simulink model "Lab6_Ris_2_20"  (Simulink 10.2)
settings: Solver=VariableStepAuto  StartTime=0.0  StopTime=10.0  RelTol=1e-3
undefined symbols (not defined in the file): dvbs2ldpc
libraries: commdigbbndam3 x5, commblkcod2 x3, commsink2 x2, commchan3 x1, commrandsrc3 x1, commutil2 x1
settings Model: Creator=Newtr  LastModifiedBy=Newtr
settings DataIOCC: SaveFormat=Dataset  SignalLoggingSaveFormat=Dataset  ReturnWorkspaceOutputs=on
settings OptimizationCC: LifeSpan=auto
settings DebuggingCC: UnderspecifiedInitializationDetection=Simplified  MergeDetectMultiDrivingBlocksExec=error  FcnCallInpInsideContextMsg=error  SFUnexpectedBacktrackingDiag=error  SFNoUnconditionalDefaultTransitionDiag=error  SFExecutionAtInitializationDiag=warning  ArithmeticOperatorsInVariantConditions=error
settings HardwareCC: ProdBitPerPointer=64  ProdBitPerSizeT=64  ProdBitPerPtrDiffT=64  ProdLargestAtomicFloat=Float  ProdIntDivRoundTo=Zero  ProdEndianess=LittleEndian  ProdWordSize=64  ProdHWDeviceType=Intel->x86-64 (Windows64)
settings ModelReferenceCC: PropagateSignalLabelsOutOfModel=on
settings SFSimCC: SimUseLocalCustomCode=on  CustomCodeUndefinedFunction=FilterOut
settings RTWCC: RTWUseLocalCustomCode=on
settings CodeAppCC: StateflowObjectComments=off
settings GRTTargetCC: TargetLangStandard=C99 (ISO)  CombineOutputUpdateFcns=on  GRTInterface=off
settings ConfigComp: CovMetricSettings=dwe  CovSaveCumulativeToWorkspaceVar=off  CovSaveSingleToWorkspaceVar=off  CovExternalEMLEnable=on

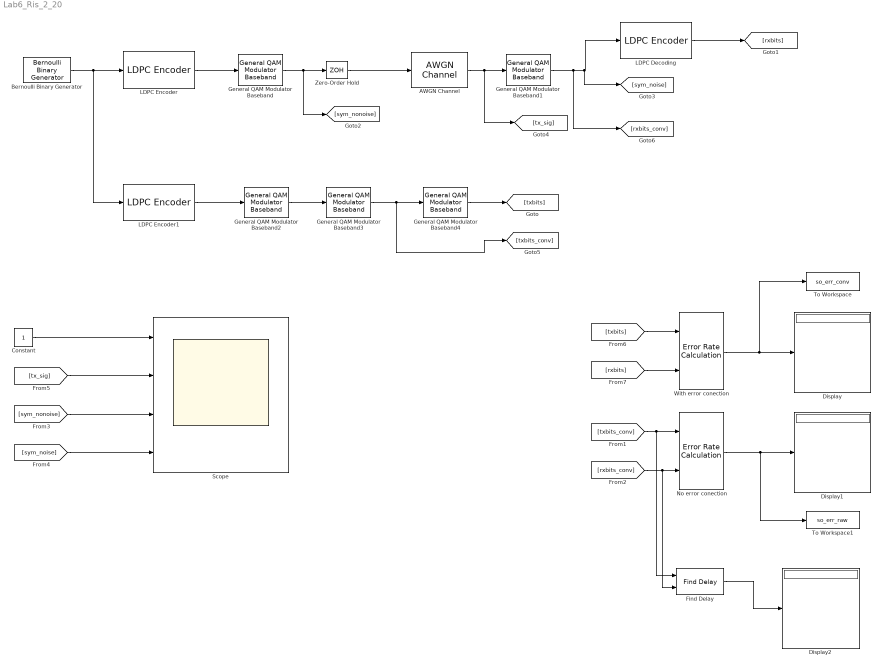
== system Lab6_Ris_2_20 ==
  AWGN Channel : commchan3/AWGN Channel  InputProcessing=Columns as channels (frame based)  seed=67  noiseMode="Signal to noise ratio  (Eb/No)"  EbNodB=10  EsNodB=10  SNRdB=10  bitsPerSym=1  Ps=1  Tsym=1  variance=1
  Bernoulli Binary Generator : commrandsrc3/Bernoulli Binary Generator  ProbabilityOfZero=0.5  SeedSource=Auto  Seed=0  SampleTime=1  SamplesPerFrame=1  OutputDataType=double  SimulateUsing=Interpreted execution
  Constant : Constant
  Display : Display
  Display1 : Display
  Display2 : Display
  Find Delay : commutil2/Find Delay  corrLength=200  chgSigOP=off  stopUpdate=off  numConstDelay=3
      settings: SourceProductBaseCode=CM
  General QAM Modulator Baseband{,1..4} (5 alike) : commdigbbndam3/General QAM Modulator Baseband  SigCon=[exp(2*pi*1i*[0:7]/8)]  outDtype=double  outWordLen=16  outUDDataType=sfix(16)  outFracLenMode=Best precision  outFracLen=15  outDataTypeStr=double  outLastDataTypeStr=double
      settings: SourceProductBaseCode=CM
  LDPC Decoding : commblkcod2/LDPC Encoder  ParityCheckMat=dvbs2ldpc(1/2)
      settings: SourceProductBaseCode=CM
  LDPC Encoder : commblkcod2/LDPC Encoder  ParityCheckMat=dvbs2ldpc(1/2)
      settings: SourceProductBaseCode=CM
  LDPC Encoder1 : commblkcod2/LDPC Encoder  ParityCheckMat=dvbs2ldpc(1/2)
      settings: SourceProductBaseCode=CM
  No error conection : commsink2/Error Rate Calculation  N=0  st_delay=0  cp_mode=Entire frame  subframe=[]  PMode=Port  WsName=ErrorVec  RsMode2=off  stop=off  numErr=100  maxBits=1e6
  Scope : Scope  NumInputPorts=4
  To Workspace : ToWorkspace  VariableName=so_err_conv  SaveFormat=Timeseries  SampleTime=-1
  To Workspace1 : ToWorkspace  VariableName=so_err_raw  SaveFormat=Timeseries  SampleTime=-1
  With error conection : commsink2/Error Rate Calculation  N=0  st_delay=0  cp_mode=Entire frame  subframe=[]  PMode=Port  WsName=ErrorVec  RsMode2=off  stop=off  numErr=100  maxBits=1e6
  Zero-Order Hold : ZeroOrderHold  SampleTime=-1
  wires:
  Bernoulli Binary Generator/1 -> LDPC Encoder1/1, LDPC Encoder/1
  LDPC Encoder/1 -> General QAM Modulator Baseband/1
  General QAM Modulator Baseband/1 -> [sym_nonoise], Zero-Order Hold/1
  Zero-Order Hold/1 -> AWGN Channel/1
  AWGN Channel/1 -> [tx_sig], General QAM Modulator Baseband1/1
  General QAM Modulator Baseband1/1 -> [rxbits_conv], [sym_noise], LDPC Decoding/1
  LDPC Decoding/1 -> [rxbits]
  LDPC Encoder1/1 -> General QAM Modulator Baseband2/1
  General QAM Modulator Baseband2/1 -> General QAM Modulator Baseband3/1
  General QAM Modulator Baseband3/1 -> [txbits_conv], General QAM Modulator Baseband4/1
  General QAM Modulator Baseband4/1 -> [txbits]
  [tx_sig] -> Scope/2
  Constant/1 -> Scope/1
  [sym_nonoise] -> Scope/3
  [sym_noise] -> Scope/4
  [txbits] -> With error conection/1
  [rxbits_conv] -> Find Delay/2, No error conection/2
  With error conection/1 -> To Workspace/1, Display/1
  [txbits_conv] -> Find Delay/1, No error conection/1
  No error conection/1 -> To Workspace1/1, Display1/1
  [rxbits] -> With error conection/2
  Find Delay/1 -> Display2/1
